simulink model "switched_simstate_hes"  (R2020a)
settings: Solver=VariableStepAuto  StartTime=0  StopTime=22  RelTol=1e-3
values from neighbouring files (symbols this model uses):
  dt = 0.001    [param_init.m]    (also in sim_switched.m = options.dt)
libraries: simulink x1
settings Model: Creator=kekatos  LastModifiedBy=kekatos
settings DataIOCC: FinalStateName=SimState  InitialState=SimState_previous  SaveFinalState=on  DSMLogging=off  ReturnWorkspaceOutputs=off

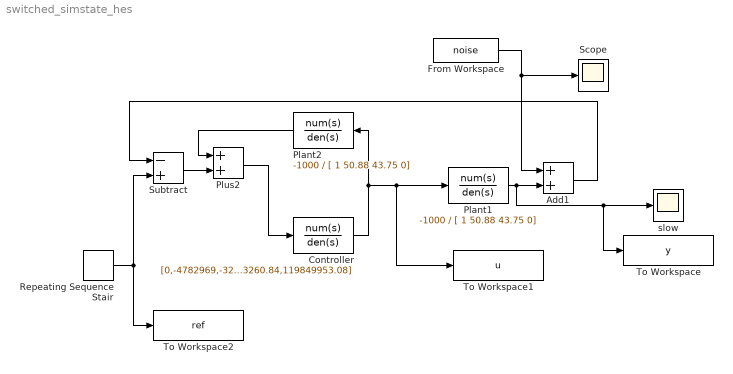
== system switched_simstate_hes ==
  Add1 : Sum
  Controller : TransferFcn  Numerator=[0,-4782969,-321787153.4913,-316286050.3938]  Denominator=[1,974.2,473260.84,119849953.08]
  From Workspace : FromWorkspace  VariableName=noise
  Plant1 : TransferFcn  Numerator=-1000  Denominator=[ 1 50.88 43.75 0]
  Plant2 : TransferFcn  Numerator=-1000  Denominator=[ 1 50.88 43.75 0]
  Plus2 : Sum
  Repeating Sequence Stair : simulink/Sources/Repeating Sequence Stair  OutValues=[1 1 1 1 1 0 0 0 0 0].'  tsamp=2  OutMin=[]  OutMax=[]  OutDataTypeStr=double  OutputDataTypeScalingMode=double  OutDataType=fixdt(0,8)  ConRadixGroup=Best Precision: Vector-wise  OutScaling=2^-12
  Scope : Scope
  Subtract : Sum  Inputs=-+
  To Workspace : ToWorkspace  VariableName=y  SaveFormat=Structure With Time  SampleTime=dt
  To Workspace1 : ToWorkspace  VariableName=u  SaveFormat=Structure With Time  SampleTime=dt
  To Workspace2 : ToWorkspace  VariableName=ref  SaveFormat=Structure With Time  SampleTime=dt
  slow : Scope
  wires:
  From Workspace/1 -> Scope/1, Add1/1
  Plant1/1 -> To Workspace/1, slow/1, Add1/2
  Repeating Sequence Stair/1 -> To Workspace2/1, Subtract/2
  Add1/1 -> Subtract/1
  Subtract/1 -> Plus2/2
  Plant2/1 -> Plus2/1
  Plus2/1 -> Controller/1
  Controller/1 -> Plant1/1, To Workspace1/1, Plant2/1
